simulink model "Wf"  (Simulink 7.3)
settings: Solver=ode45  StartTime=0.0  StopTime=4.0  RelTol=1e-3
libraries: simulink x2
settings Model: Creator=SAINQUAKE  LastModifiedBy=SAINQUAKE

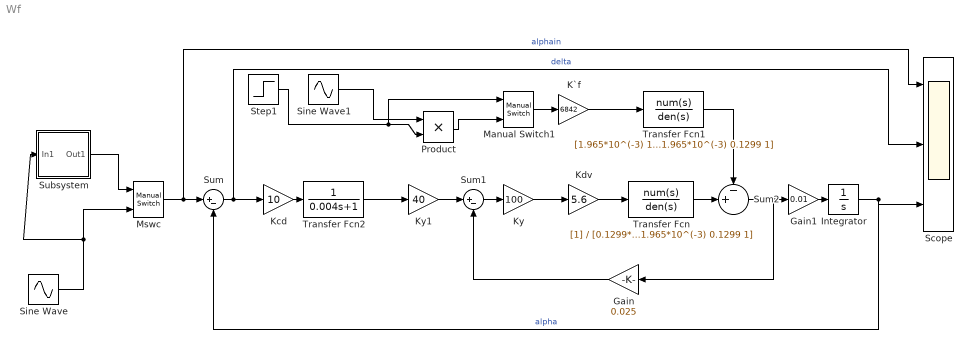
== system Wf ==
  Gain : Gain  Gain=0.025  ParameterDataType=fixdt(1, 16)  ParameterScaling=2^0  OutDataType=fixdt(1, 16)  OutScaling=2^0
  Gain1 : Gain  Gain=0.01  ParameterDataType=fixdt(1, 16)  ParameterScaling=2^0  OutDataType=fixdt(1, 16)  OutScaling=2^0
  Integrator : Integrator
  K`f : Gain  Gain=6842  ParameterDataType=fixdt(1, 16)  ParameterScaling=2^0  OutDataType=fixdt(1, 16)  OutScaling=2^0
  Kcd : Gain  Gain=10  ParameterDataType=fixdt(1, 16)  ParameterScaling=2^0  OutDataType=fixdt(1, 16)  OutScaling=2^0
  Kdv : Gain  Gain=5.6  ParameterDataType=fixdt(1, 16)  ParameterScaling=2^0  OutDataType=fixdt(1, 16)  OutScaling=2^0
  Ky : Gain  Gain=100  ParameterDataType=fixdt(1, 16)  ParameterScaling=2^0  OutDataType=fixdt(1, 16)  OutScaling=2^0
  Ky1 : Gain  Gain=40  ParameterDataType=fixdt(1, 16)  ParameterScaling=2^0  OutDataType=fixdt(1, 16)  OutScaling=2^0
  Manual Switch1 : simulink/Signal Routing/Manual Switch  SystemSampleTime=-1  sw=0  action=0  varsize=off
  Mswc : simulink/Signal Routing/Manual Switch  SystemSampleTime=-1  sw=0  action=0  varsize=off
  Product : Product  OutDataType=fixdt(1, 16)  OutScaling=2^0  RndMeth=Zero
  Scope : Scope  NumInputPorts=3
      settings: YMin=-5~-5~-5  YMax=5~5~5
  Sine Wave : Sin  Amplitude=1  Bias=0  Frequency=10  Phase=0  Samples=10  SampleTime=0  Offset=0
  Sine Wave1 : Sin  Amplitude=1.4  Bias=0  Frequency=2  Phase=0  Samples=10  SampleTime=0  Offset=0
  Step1 : Step  After=1.4  SampleTime=0
  Subsystem : Subsystem
  Sum : Sum  Inputs=|+-  OutDataType=fixdt(1, 16)  OutScaling=2^0
  Sum1 : Sum  Inputs=|+-  OutDataType=fixdt(1, 16)  OutScaling=2^0
  Sum2 : Sum  Inputs=-+|  OutDataType=fixdt(1, 16)  OutScaling=2^0
  Transfer Fcn : TransferFcn  Denominator=[0.1299*1.965*10^(-3) 0.1299 1]
  Transfer Fcn1 : TransferFcn  Numerator=[1.965*10^(-3) 1]  Denominator=[0.1299*1.965*10^(-3) 0.1299 1]
  Transfer Fcn2 : TransferFcn  Denominator=[0.004 1]
  wires:
  Mswc/1 -> Sum/1, Scope/1  "alphain"
  Subsystem/1(Out1) -> Mswc/1
  Sum/1 -> Scope/2, Kcd/1  "delta"
  Sum1/1 -> Ky/1
  Transfer Fcn/1 -> Sum2/2
  Sum2/1 -> Gain/1, Gain1/1
  Integrator/1 -> Sum/2, Scope/3  "alpha"
  Gain/1 -> Sum1/2
  Gain1/1 -> Integrator/1
  Ky1/1 -> Sum1/1
  Sine Wave/1 -> Mswc/2, Subsystem/1(In1)
  Transfer Fcn1/1 -> Sum2/1
  Kdv/1 -> Transfer Fcn/1
  K`f/1 -> Transfer Fcn1/1
  Manual Switch1/1 -> K`f/1
  Kcd/1 -> Transfer Fcn2/1
  Transfer Fcn2/1 -> Ky1/1
  Ky/1 -> Kdv/1
  Product/1 -> Manual Switch1/2
  Sine Wave1/1 -> Product/1
  Step1/1 -> Product/2, Manual Switch1/1

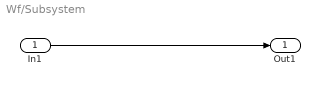
== system Wf/Subsystem ==
  In1 : Inport  OutDataType=fixdt(1, 16)  OutScaling=2^0
  Out1 : Outport  OutDataType=fixdt(1, 16)  OutScaling=2^0
  wires:
  In1/1 -> Out1/1
